simulink library "PMPNetZeroSpoolingController_ul"  (R2018b)
settings: Solver=VariableStepAuto  StartTime=0.0  StopTime=10.0  RelTol=1e-3
undefined symbols (not defined in the file or in its folder): env, pstrat, Ten
libraries: simulink x8, stopwatch_ul x1, runningAvg_ul x1
settings Model: Creator=James Reed  LastModifiedBy=mcobb

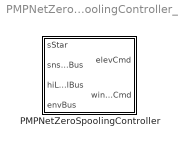
== system PMPNetZeroSpoolingController_ul ==
  PMPNetZeroSpoolingController : Subsystem  mask{reelInDefl=23, reelOutDefl=0}
      mask prompts: reelInDefl "Reel In Elevator Deflection [deg]"; reelOutDefl "Reel Out Elevator Deflection [deg]"
      mask TypeOptions reelInDefl: ReelInElevDefl/Value
      mask TypeOptions reelOutDefl: ReelOutElevDefl/Value

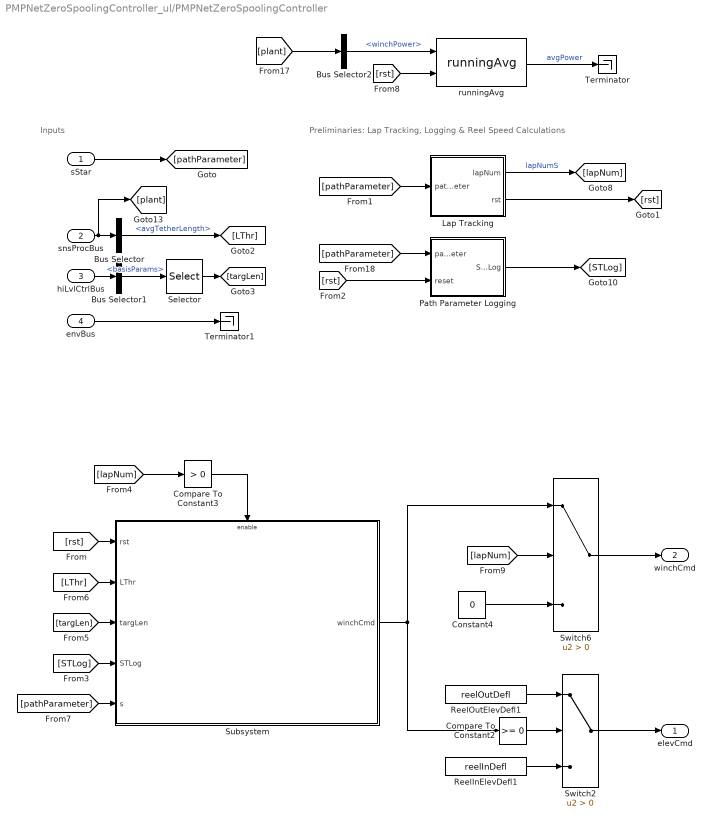
== system PMPNetZeroSpoolingController_ul/PMPNetZeroSpoolingController ==
  note: Inputs
  note: Preliminaries: Lap Tracking, Logging & Reel Speed Calculations
  "sStar " : Inport
  snsProcBus : Inport  Port=2  OutDataTypeStr=Bus: sensorsProcessingBus
  hiLvlCtrlBus : Inport  Port=3  OutDataTypeStr=Bus: hiLvlCtrlBus
  envBus : Inport  Port=4  OutDataTypeStr=Bus: envBus
  Bus Selector : BusSelector  OutputSignals=avgTetherLength
  Bus Selector1 : BusSelector  OutputSignals=basisParams
  Bus Selector2 : BusSelector  OutputSignals=winchPower
  Compare To Constant2 : simulink/Logic and Bit Operations/Compare To Constant  relop=>=  const=0  OutDataTypeStr=boolean
  Compare To Constant3 : simulink/Logic and Bit Operations/Compare To Constant  relop=>  const=0  OutDataTypeStr=boolean
  Constant4 : Constant  Value=0
  Lap Tracking : Subsystem
  Path Parameter Logging : Subsystem
  ReelInElevDefl1 : Constant  Value=reelInDefl
  ReelOutElevDefl1 : Constant  Value=reelOutDefl
  Selector : Selector  InputPortWidth=5  IndexOptions=Index vector (dialog)  Indices=5  OutputSizes=1
  Subsystem : Subsystem
  Switch2 : Switch  Criteria=u2 > Threshold
  Switch6 : Switch  Criteria=u2 > Threshold
  Terminator : Terminator
  Terminator1 : Terminator
  runningAvg : runningAvg_ul/runningAvg  SystemSampleTime=-1
  elevCmd : Outport
  "winchCmd " : Outport  Port=2
  wires:
  hiLvlCtrlBus/1 -> Bus Selector1/1
  "sStar "/1 -> [pathParameter]
  Bus Selector/1 -> [LThr]  "<avgTetherLength>"
  [pathParameter] -> Path Parameter Logging/1(pathParameter)
  [rst] -> Path Parameter Logging/2(reset)
  Path Parameter Logging/1(SVsTLog) -> [STLog]
  envBus/1 -> Terminator1/1
  [pathParameter] -> Lap Tracking/1(pathParameter)
  Lap Tracking/1(lapNum) -> [lapNum]  "lapNumS"
  Lap Tracking/2(rst) -> [rst]
  Bus Selector1/1 -> Selector/1  "<basisParams>"
  Selector/1 -> [targLen]
  ReelInElevDefl1/1 -> Switch2/3
  ReelOutElevDefl1/1 -> Switch2/1
  [rst] -> runningAvg/2
  Bus Selector2/1 -> runningAvg/1  "<winchPower>"
  runningAvg/1 -> Terminator/1  "avgPower"
  snsProcBus/1 -> [plant], Bus Selector/1
  [plant] -> Bus Selector2/1
  Compare To Constant2/1 -> Switch2/2
  Switch2/1 -> elevCmd/1
  Compare To Constant3/1 -> Subsystem/Enable
  Constant4/1 -> Switch6/3
  [lapNum] -> Switch6/2
  Switch6/1 -> "winchCmd "/1
  [lapNum] -> Compare To Constant3/1
  Subsystem/1(winchCmd) -> Compare To Constant2/1, Switch6/1
  [rst] -> Subsystem/1(rst)
  [STLog] -> Subsystem/4(STLog)
  [targLen] -> Subsystem/3(targLen)
  [LThr] -> Subsystem/2(LThr)
  [pathParameter] -> Subsystem/5(s)

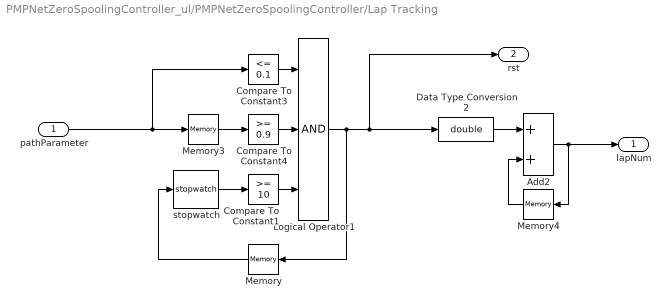
== system PMPNetZeroSpoolingController_ul/PMPNetZeroSpoolingController/Lap Tracking ==
  pathParameter : Inport
  Add2 : Sum
  Compare To Constant1 : simulink/Logic and Bit Operations/Compare To Constant  relop=>=  const=10  OutDataTypeStr=boolean
  Compare To Constant3 : simulink/Logic and Bit Operations/Compare To Constant  relop=<=  const=0.1  OutDataTypeStr=boolean
  Compare To Constant4 : simulink/Logic and Bit Operations/Compare To Constant  relop=>=  const=0.9  OutDataTypeStr=boolean
  Data Type Conversion2 : DataTypeConversion  OutDataTypeStr=double
  Logical Operator1 : Logic  Inputs=3  AllPortsSameDT=off  OutDataTypeStr=boolean
  Memory : Memory  InitialCondition=false
  Memory3 : Memory
  Memory4 : Memory
  stopwatch : stopwatch_ul/stopwatch  SystemSampleTime=-1
  lapNum : Outport
  rst : Outport  Port=2
  wires:
  Compare To Constant3/1 -> Logical Operator1/1
  Memory3/1 -> Compare To Constant4/1
  Data Type Conversion2/1 -> Add2/1
  Memory4/1 -> Add2/2
  Add2/1 -> lapNum/1, Memory4/1
  Compare To Constant4/1 -> Logical Operator1/2
  pathParameter/1 -> Compare To Constant3/1, Memory3/1
  Compare To Constant1/1 -> Logical Operator1/3
  stopwatch/1 -> Compare To Constant1/1
  Memory/1 -> stopwatch/1
  Logical Operator1/1 -> Memory/1, rst/1, Data Type Conversion2/1

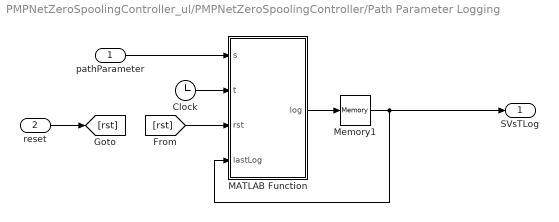
== system PMPNetZeroSpoolingController_ul/PMPNetZeroSpoolingController/Path Parameter Logging ==
  pathParameter : Inport
  reset : Inport  Port=2
  Clock : Clock
  MATLAB Function : MATLAB Function  TreatAsAtomicUnit=on
  Memory1 : Memory  InitialCondition=zeros(1000,2)
  SVsTLog : Outport
  wires:
  MATLAB Function/1(log) -> Memory1/1
  reset/1 -> [rst]
  pathParameter/1 -> MATLAB Function/1(s)
  Clock/1 -> MATLAB Function/2(t)
  Memory1/1 -> SVsTLog/1, MATLAB Function/4(lastLog)
  [rst] -> MATLAB Function/3(rst)

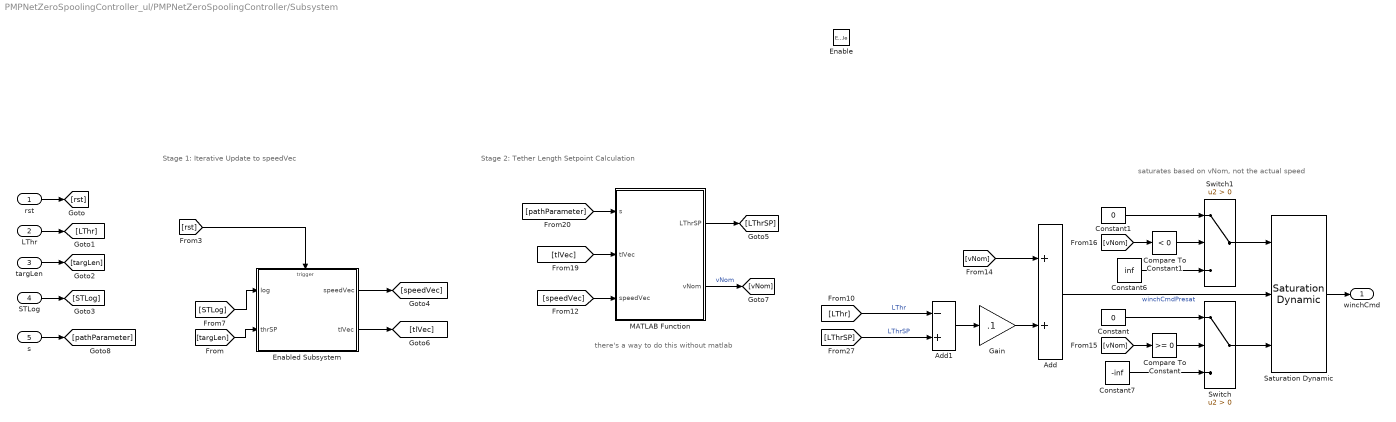
== system PMPNetZeroSpoolingController_ul/PMPNetZeroSpoolingController/Subsystem ==
  note: there's a way to do this without matlab
  note: saturates based on vNom, not the actual speed
  note: Stage 1: Iterative Update to speedVec
  note: Stage 2: Tether Length Setpoint Calculation
  rst : Inport
  LThr : Inport  Port=2
  targLen : Inport  Port=3
  STLog : Inport  Port=4
  s : Inport  Port=5
  Enable : EnablePort
  Add : Sum
  Add1 : Sum  Inputs=-+
  Compare To Constant : simulink/Logic and Bit Operations/Compare To Constant  relop=>=  const=0  OutDataTypeStr=boolean
  Compare To Constant1 : simulink/Logic and Bit Operations/Compare To Constant  relop=<  const=0  OutDataTypeStr=boolean
  Constant : Constant  Value=0
  Constant1 : Constant  Value=0
  Constant6 : Constant  Value=inf
  Constant7 : Constant  Value=-inf
  Enabled Subsystem : Subsystem  TreatAsAtomicUnit=on  mask{guess=mean(mean(Ten)), Ten=Ten, pstrat=pstrat, speedRange=norm(env.water.flowVec.Value)*.4}
      mask prompts: guess "Initial costate guess"; Ten "1000x1000 Ten Surf"; pstrat "P vs Strat Matrix"; speedRange "Spooling Sat. Limits"
  Gain : Gain  Gain=.1
  MATLAB Function : MATLAB Function  TreatAsAtomicUnit=on
  Saturation Dynamic : simulink/Discontinuities/Saturation Dynamic  OutMin=[]  OutMax=[]  OutDataTypeStr=Inherit: Same as second input  OutDataType=fixdt(1, 16)  OutScaling=2^-10  DoSatur=off
  Switch : Switch  Criteria=u2 > Threshold
  Switch1 : Switch  Criteria=u2 > Threshold
  winchCmd : Outport  InitialOutput=[0]
  wires:
  [LThr] -> Add1/1  "LThr"
  [rst] -> Enabled Subsystem/Trigger
  Constant7/1 -> Switch/3
  Enabled Subsystem/2(tlVec) -> [tlVec]
  Enabled Subsystem/1(speedVec) -> [speedVec]
  Saturation Dynamic/1 -> winchCmd/1
  Constant/1 -> Switch/1
  Add/1 -> Saturation Dynamic/2  "winchCmdPresat"
  Constant6/1 -> Switch1/3
  Constant1/1 -> Switch1/1
  MATLAB Function/1(LThrSP) -> [LThrSP]
  MATLAB Function/2(vNom) -> [vNom]  "vNom"
  Switch/1 -> Saturation Dynamic/3
  [LThrSP] -> Add1/2  "LThrSP"
  [vNom] -> Compare To Constant/1
  [vNom] -> Add/1
  Compare To Constant/1 -> Switch/2
  [pathParameter] -> MATLAB Function/1(s)
  Compare To Constant1/1 -> Switch1/2
  Switch1/1 -> Saturation Dynamic/1
  [vNom] -> Compare To Constant1/1
  [STLog] -> Enabled Subsystem/1(log)
  Gain/1 -> Add/2
  Add1/1 -> Gain/1
  [tlVec] -> MATLAB Function/2(tlVec)
  [speedVec] -> MATLAB Function/3(speedVec)
  rst/1 -> [rst]
  LThr/1 -> [LThr]
  STLog/1 -> [STLog]
  s/1 -> [pathParameter]
  targLen/1 -> [targLen]
  [targLen] -> Enabled Subsystem/2("thrSP ")

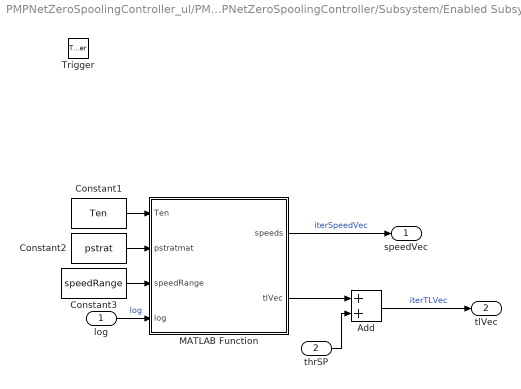
== system PMPNetZeroSpoolingController_ul/PMPNetZeroSpoolingController/Subsystem/Enabled Subsystem ==
  log : Inport
  "thrSP " : Inport  Port=2
  Trigger : TriggerPort  VariantControl=Variant  PortDimensions=1
  Add : Sum
  Constant1 : Constant  Value=Ten
  Constant2 : Constant  Value=pstrat
  Constant3 : Constant  Value=speedRange
  MATLAB Function : MATLAB Function  TreatAsAtomicUnit=on
  speedVec : Outport
  tlVec : Outport  Port=2
  wires:
  Constant3/1 -> MATLAB Function/3(speedRange)
  MATLAB Function/1(speeds) -> speedVec/1  "iterSpeedVec"
  Constant1/1 -> MATLAB Function/1(Ten)
  log/1 -> MATLAB Function/4(log)  "log"
  Constant2/1 -> MATLAB Function/2(pstratmat)
  MATLAB Function/2(tlVec) -> Add/1
  "thrSP "/1 -> Add/2
  Add/1 -> tlVec/1  "iterTLVec"

== matlab function PMPNetZeroSpoolingController_ul/PMPNetZeroSpoolingController/Subsystem/Enabled Subsystem/MATLAB Function ==
  data: Ten input; pstratmat input; speeds output; speedRange input; log input; tlVec output
function [speeds, tlVec] = fcn(Ten, pstratmat, speedRange, log)
cleanLog = log( and( and(log(:,1)~=0,log(:,2)~=0),and(~isnan(log(:,1)),~isnan(log(:,2))) ),:);
% deltaVec=mean(diff(cleanLog(:,1))./diff(cleanLog(:,2)));
evenlog=[linspace(0,1,1000)',interp1(cleanLog(:,1),cleanLog(:,2),linspace(0,1,1000)','linear','extrap')];
diffTime = diff(evenlog(:,2)); 
timesteps = .5*([diffTime; diffTime(end)] + [diffTime(1); diffTime]); %averages left and right timestep lengths for each data point.

ps = linspace(min(min(Ten)),max(max(Ten)),100)';
deltaLest = pstratmat*timesteps;
[~,minind]=min(abs(deltaLest));
deltaLinterp = linspace(deltaLest(minind-1),deltaLest(minind+1),100)';
pinterp=linspace(ps(minind-1),ps(minind+1),100)';
[~,minind2]=min(abs(deltaLinterp));
p=pinterp(minind2);


xopts=linspace(speedRange(1),speedRange(2),max(size(Ten)));
n=1000;
% speeds = zeros(2*max(size(Ten)),1);
speeds = zeros(n,1);
% for ii = 1:2*max(size(Ten))
for ii = 1:n
    iidbl=(1000/n)*ii;
    %     hamil = @(x) (p-Ten(ii,xopts==x)).*x;
    perc=iidbl-floor(iidbl);
    currTen=((1-perc)*Ten(max(floor(iidbl),1),:)) + (perc*Ten(ceil(iidbl),:));
    hamil = @(x) (p-interp1(xopts,currTen,x)).*x;
    [~,bestind]=min(hamil(xopts));
    bestx=xopts(bestind);
    
    step=xopts(2)-xopts(1);
    lbnd = max(xopts(1),bestx-step);
    rbnd = min(xopts(end),bestx+step);
    tau = 1-.38197;
    for i=1:5
        x1=((1-tau)*rbnd)+(tau*lbnd);
        x2=((1-tau)*lbnd)+(tau*rbnd);
        f1=hamil(x1);
        f2=hamil(x2);
        if f1>=f2
            lbnd=x1;
        else
            rbnd=x2;
        end
    end
    bestx=(lbnd+rbnd)/2;
    speeds(ii)=bestx;
end
if isempty(isnan(cleanLog(:,1)))
    err=1;
end

lengthSteps=speeds(:).*timesteps(:);
tlVec=cumsum(lengthSteps);

== matlab function PMPNetZeroSpoolingController_ul/PMPNetZeroSpoolingController/Path Parameter Logging/MATLAB Function ==
  data: s input; log output; t input; rst input; lastLog input
function log = fcn(s,t,rst,lastLog)
% function that logs the path position and time into a matrix
% [pathPosition,t]
if rst
    lastLog = nan(1000,2);
end
log = lastLog;
idx = min([max([round(s*1000),1]),1000]);
log(idx,1) = s;
log(idx,2) = t;

== matlab function PMPNetZeroSpoolingController_ul/PMPNetZeroSpoolingController/Subsystem/MATLAB Function ==
  data: s input; LThrSP output; tlVec input; speedVec input; vNom output
function [LThrSP,vNom] = fcn(s,tlVec,speedVec)
    LThrSP=interp1(linspace(0,1,1000),tlVec,s);
    vNom=interp1(linspace(0,1,1000),speedVec,s);
